simulink library "Ann1Path"  (R2022b)
settings: Solver=VariableStepAuto  StartTime=0.0  StopTime=10.0  RelTol=1e-3
undefined symbols (not defined in the file or in its folder): ModelSettings
libraries: PoolIir x2, FeaturePath x2, TunableDelayBtc x1, AnnGainCalcBtc x1, SelectiveChannelMuteBtc x1, RouterBtc x1, AnnSteeringBtc x1, AnnVncBtc x1, AnnVolumeBtc x1, HandyTextFile x1, AnnLimiterBtc x1, AsdRouterBtc x1
settings Model: Creator=st51187  LastModifiedBy=st51187

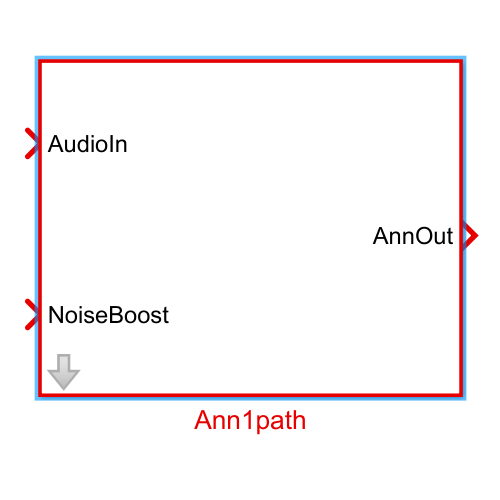
[thumbnail: Simulink's stored preview of the top-level diagram]
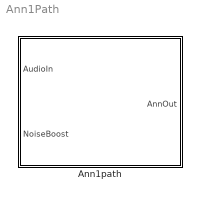
== system Ann1Path ==
  Ann1path : Subsystem  TreatAsAtomicUnit=on  mask{Config=ModelSettings.Ann1path}
      mask prompts: Config "Ann1pathConfig"
      mask init:
      | blkh=gcbh;
      | Config=BTConfig.Assert(blkh,Config);
      | 
      | Config.Validate();
      | Config.DoMaskInit(blkh);
      settings: LibrarySourceBlock=Ann1Path/Ann1path

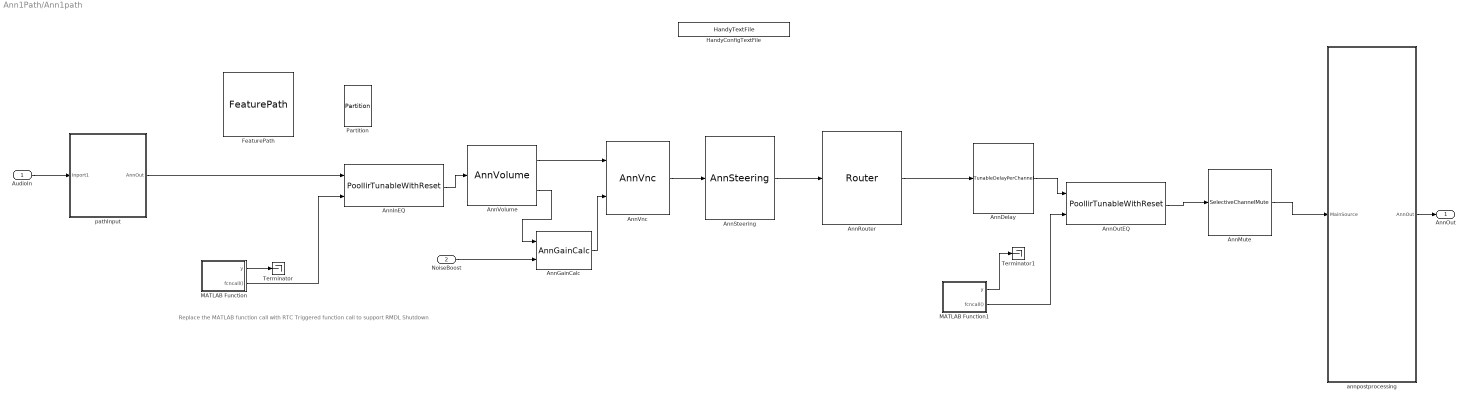
== system Ann1Path/Ann1path ==
  note: Replace the MATLAB function call with RTC Triggered function call to support RMDL Shutdown
  AudioIn : Inport
  NoiseBoost : Inport  Port=2
  AnnDelay : TunableDelayBtc/TunableDelayPerChannel  Config=Config.AnnDelay  FeatureName=AnnDelay
      settings: SourceProductName=Bose Blocklib
  AnnGainCalc : AnnGainCalcBtc/AnnGainCalc  Config=Config.AnnGainCalc  FeatureName=AnnGainCalc
      settings: SourceProductName=Bose Blocklib
  AnnInEQ : PoolIir/PoolIirTunableWithReset  FeatureName=AnnInEQ  Config=Config.AnnInEQ
  AnnMute : SelectiveChannelMuteBtc/SelectiveChannelMute  Config=Config.AnnMute  FeatureName=AnnMute
      settings: SourceProductName=Bose Blocklib
  AnnOutEQ : PoolIir/PoolIirTunableWithReset  FeatureName=AnnOutEQ  Config=Config.AnnOutEQ
  AnnRouter : RouterBtc/Router  Config=Config.AnnRouter  FeatureName=AnnRouter
      settings: SourceProductName=Bose Blocklib
  AnnSteering : AnnSteeringBtc/AnnSteering  Config=Config.AnnSteering  FeatureName=AnnSteering
      settings: SourceProductName=Bose Blocklib
  AnnVnc : AnnVncBtc/AnnVnc  Config=Config.AnnVnc  FeatureName=AnnVnc
      settings: SourceProductName=Bose Blocklib
  AnnVolume : AnnVolumeBtc/AnnVolume  FeatureName=AnnVolume  Config=Config.AnnVolume  TriggerInit=[775 180 890 280]
      settings: SourceProductName=Bose Blocklib
  FeaturePath : FeaturePath/FeaturePath  FeatureName=Announcements  IsGroup=off  GroupNumber=0  IsModule=on  TriggerInit=[370 59 485 166]
      settings: SourceProductName=Bose Talaria
  HandyConfigTextFile : HandyTextFile/HandyTextFile  TemplateSource=Config  FileSuffix=File  OpenDialogOnLoad=off  UseThisBlockName=off  AddGrandParentNamePrefix=off  TheDefaultText=% $(FILENAME) $(PREFIX) $(SUFFIX)  ShowInLibBrowser=on
      settings: SourceProductName=Bose Talaria
  MATLAB Function : MATLAB Function  TreatAsAtomicUnit=on
  MATLAB Function1 : MATLAB Function  TreatAsAtomicUnit=on
  Partition : FeaturePath/Partition  PartitionNumber=0  TriggerInit=[570 81 615 149]
      settings: SourceProductName=Bose Talaria
  Terminator : Terminator
  Terminator1 : Terminator
  annpostprocessing : Subsystem  TreatAsAtomicUnit=on
      settings: RTWSystemCode=Nonreusable function  RTWFcnNameOpts=Use subsystem name  RTWFileNameOpts=Use subsystem name  FunctionWithSeparateData=on
  pathInput : Subsystem
  AnnOut : Outport
  wires:
  MATLAB Function1/2(fcncall()) -> AnnOutEQ/2
  AnnDelay/1 -> AnnOutEQ/1
  AnnRouter/1 -> AnnDelay/1
  AnnOutEQ/1 -> AnnMute/1
  AnnInEQ/1 -> AnnVolume/1
  annpostprocessing/1(AnnOut) -> AnnOut/1
  pathInput/1(AnnOut) -> AnnInEQ/1
  AnnSteering/1 -> AnnRouter/1
  AnnGainCalc/1 -> AnnVnc/2
  AnnVolume/2 -> AnnGainCalc/1
  AnnVnc/1 -> AnnSteering/1
  AnnMute/1 -> annpostprocessing/1(MainSource)
  AudioIn/1 -> pathInput/1(Inport1)
  AnnVolume/1 -> AnnVnc/1
  NoiseBoost/1 -> AnnGainCalc/2
  MATLAB Function/2(fcncall()) -> AnnInEQ/2
  MATLAB Function/1(y) -> Terminator/1
  MATLAB Function1/1(y) -> Terminator1/1

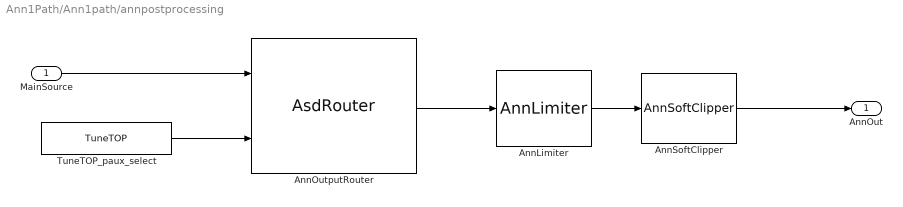
== system Ann1Path/Ann1path/annpostprocessing ==
  MainSource : Inport
  AnnLimiter : AnnLimiterBtc/AnnLimiter  Config=Config.AnnLimiter  FeatureName=AnnLimiter
      settings: SourceProductName=Bose Blocklib
  AnnOutputRouter : AsdRouterBtc/AsdRouter  Config=Config.AnnOutputRouter  FeatureName=AnnOutputRouter
      settings: SourceProductName=Bose Blocklib
  AnnSoftClipper : AnnSoftClipperBtc/AnnSoftClipper  Config=Config.AnnSoftClipper  FeatureName=AnnSoftClipper
      settings: SourceProductName=Bose Blocklib
  TuneTOP_paux_select : TuneVar/TuneTOP  TriggerInit=[185 194 315 226]  TopName=AuxSelect  TuneName=AuxSelect  DataType=int32  TunabilityNumber=1  MinValue=[]  MaxValue=[]  BankNumber=0  PreOverlay=false  PostOverlay=false  UseSameName=on  MaskValue=Config.aux_select
      settings: SourceProductName=Bose Talaria
  AnnOut : Outport
  wires:
  TuneTOP_paux_select/1 -> AnnOutputRouter/2
  AnnSoftClipper/1 -> AnnOut/1
  AnnLimiter/1 -> AnnSoftClipper/1
  AnnOutputRouter/1 -> AnnLimiter/1
  MainSource/1 -> AnnOutputRouter/1

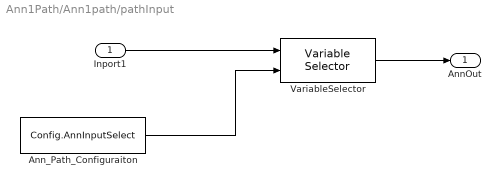
== system Ann1Path/Ann1path/pathInput ==
  Inport1 : Inport
  Ann_Path_Configuraiton : Constant  Value=Config.AnnInputSelect  VectorParams1D=off  OutDataTypeStr=single
  VariableSelector : dspindex/Variable Selector  NumInputs=1  rowsOrCols=Columns  IdxMode=Variable  Elements=[1:2]  ZerOneIdxMode=One-based  errmode=Clip Index  FillMode=off  FillValues=0
  AnnOut : Outport  VectorParamsAs1DForOutWhenUnconnected=off
  wires:
  Inport1/1 -> VariableSelector/1
  Ann_Path_Configuraiton/1 -> VariableSelector/2
  VariableSelector/1 -> AnnOut/1

== matlab function Ann1Path/Ann1path/MATLAB Function ==
  data: y output
  events: fcncall output FUNCTION_CALL_EVENT
function y = fcn

y = true;

== matlab function Ann1Path/Ann1path/MATLAB Function1 ==
  data: y output
  events: fcncall output FUNCTION_CALL_EVENT
function y = fcn

y = true;
